simulink model "ACC_Project"  (R2020a)
settings: Solver=FixedStepDiscrete  StartTime=0.0  StopTime=10.0  FixedStep=0.01  RelTol=1e-3
settings Model: DataDictionary=ACC_Project_SLDD.sldd  EnableAccessToBaseWorkspace=off  Creator=todka  LastModifiedBy=todka
settings OptimizationCC: DefaultParameterBehavior=Inlined  EnhancedBackFolding=on  PassReuseOutputArgsAs=Individual arguments  ZeroExternalMemoryAtStartup=off  ZeroInternalMemoryAtStartup=off  OptimizeBlockOrder=speed  DifferentSizesBufferReuse=on  OptimizationCustomize=off  EfficientTunableParamExpr=on
settings DebuggingCC: SignalInfNanChecking=error  CheckMatrixSingularityMsg=error  IntegerOverflowMsg=error  ParameterTunabilityLossMsg=error  UniqueDataStoreMsg=error  StrictBusMsg=ErrorOnBusTreatedAsVector  IntegerSaturationMsg=error
settings SFSimCC: MATLABDynamicMemAlloc=off
settings RTWCC: SystemTargetFile=ert.tlc  TemplateMakefile=ert_default_tmf  GenerateReport=on
settings CodeAppCC: ForceParamTrailComments=on  IgnoreCustomStorageClasses=off  OperatorAnnotations=on  SimulinkDataObjDesc=on  SFDataObjDesc=on  InsertBlockDesc=on
settings ERTTargetCC: TargetLangStandard=C99 (ISO)  GenerateSampleERTMain=on  InlinedParameterPlacement=NonHierarchical  ERTCustomFileTemplate=example_file_process.tlc
settings ConfigComp: CovMetricSettings=dcmwe

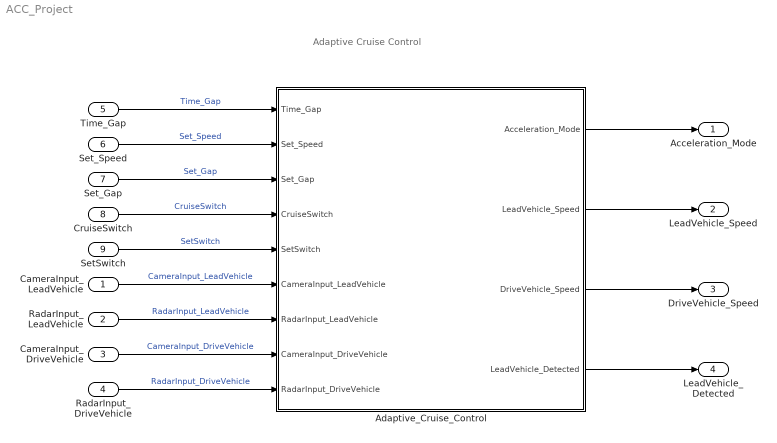
== system ACC_Project ==
  note: Adaptive Cruise Control
  CameraInput_LeadVehicle : Inport
  RadarInput_LeadVehicle : Inport  Port=2
  CameraInput_DriveVehicle : Inport  Port=3
  RadarInput_DriveVehicle : Inport  Port=4
  Time_Gap : Inport  Port=5
  Set_Speed : Inport  Port=6
  Set_Gap : Inport  Port=7
  CruiseSwitch : Inport  Port=8
  SetSwitch : Inport  Port=9
  Adaptive_Cruise_Control : Subsystem
  Acceleration_Mode : Outport
  LeadVehicle_Speed : Outport  Port=2
  DriveVehicle_Speed : Outport  Port=3
  LeadVehicle_Detected : Outport  Port=4
  wires:
  Time_Gap/1 -> Adaptive_Cruise_Control/1(Time_Gap)  "Time_Gap"
  Set_Speed/1 -> Adaptive_Cruise_Control/2(Set_Speed)  "Set_Speed"
  Set_Gap/1 -> Adaptive_Cruise_Control/3(Set_Gap)  "Set_Gap"
  CruiseSwitch/1 -> Adaptive_Cruise_Control/4(CruiseSwitch)  "CruiseSwitch"
  SetSwitch/1 -> Adaptive_Cruise_Control/5(SetSwitch)  "SetSwitch"
  CameraInput_LeadVehicle/1 -> Adaptive_Cruise_Control/6(CameraInput_LeadVehicle)  "CameraInput_LeadVehicle"
  RadarInput_LeadVehicle/1 -> Adaptive_Cruise_Control/7(RadarInput_LeadVehicle)  "RadarInput_LeadVehicle"
  CameraInput_DriveVehicle/1 -> Adaptive_Cruise_Control/8(CameraInput_DriveVehicle)  "CameraInput_DriveVehicle"
  RadarInput_DriveVehicle/1 -> Adaptive_Cruise_Control/9(RadarInput_DriveVehicle)  "RadarInput_DriveVehicle"
  Adaptive_Cruise_Control/1(Acceleration_Mode) -> Acceleration_Mode/1
  Adaptive_Cruise_Control/2(LeadVehicle_Speed) -> LeadVehicle_Speed/1
  Adaptive_Cruise_Control/3(DriveVehicle_Speed) -> DriveVehicle_Speed/1
  Adaptive_Cruise_Control/4(LeadVehicle_Detected) -> LeadVehicle_Detected/1

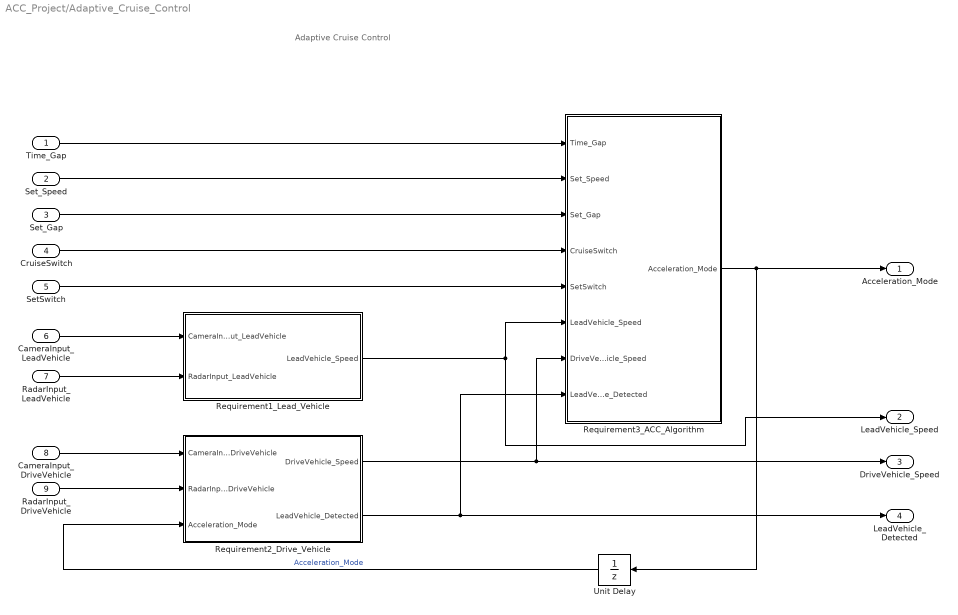
== system ACC_Project/Adaptive_Cruise_Control ==
  note: Adaptive Cruise Control
  Time_Gap : Inport
  Set_Speed : Inport  Port=2
  Set_Gap : Inport  Port=3
  CruiseSwitch : Inport  Port=4
  SetSwitch : Inport  Port=5
  CameraInput_LeadVehicle : Inport  Port=6
  RadarInput_LeadVehicle : Inport  Port=7
  CameraInput_DriveVehicle : Inport  Port=8
  RadarInput_DriveVehicle : Inport  Port=9
  Requirement1_Lead_Vehicle : Subsystem
  Requirement2_Drive_Vehicle : Subsystem
  Requirement3_ACC_Algorithm : Subsystem
  Unit Delay : UnitDelay  SampleTime=-1  HasFrameUpgradeWarning=on
  Acceleration_Mode : Outport
  LeadVehicle_Speed : Outport  Port=2
  DriveVehicle_Speed : Outport  Port=3
  LeadVehicle_Detected : Outport  Port=4
  wires:
  Requirement2_Drive_Vehicle/2(LeadVehicle_Detected) -> Requirement3_ACC_Algorithm/8(LeadVehicle_Detected), LeadVehicle_Detected/1
  CruiseSwitch/1 -> Requirement3_ACC_Algorithm/4(CruiseSwitch)
  Requirement1_Lead_Vehicle/1(LeadVehicle_Speed) -> LeadVehicle_Speed/1, Requirement3_ACC_Algorithm/6(LeadVehicle_Speed)
  SetSwitch/1 -> Requirement3_ACC_Algorithm/5(SetSwitch)
  Time_Gap/1 -> Requirement3_ACC_Algorithm/1(Time_Gap)
  Set_Gap/1 -> Requirement3_ACC_Algorithm/3(Set_Gap)
  RadarInput_LeadVehicle/1 -> Requirement1_Lead_Vehicle/2(RadarInput_LeadVehicle)
  Set_Speed/1 -> Requirement3_ACC_Algorithm/2(Set_Speed)
  Requirement2_Drive_Vehicle/1(DriveVehicle_Speed) -> DriveVehicle_Speed/1, Requirement3_ACC_Algorithm/7(DriveVehicle_Speed)
  CameraInput_DriveVehicle/1 -> Requirement2_Drive_Vehicle/1(CameraInput_DriveVehicle)
  CameraInput_LeadVehicle/1 -> Requirement1_Lead_Vehicle/1(CameraInput_LeadVehicle)
  RadarInput_DriveVehicle/1 -> Requirement2_Drive_Vehicle/2(RadarInput_DriveVehicle)
  Requirement3_ACC_Algorithm/1(Acceleration_Mode) -> Unit Delay/1, Acceleration_Mode/1
  Unit Delay/1 -> Requirement2_Drive_Vehicle/3(Acceleration_Mode)  "Acceleration_Mode"

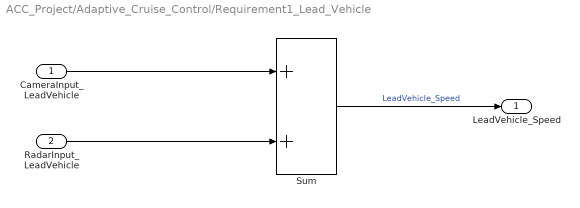
== system ACC_Project/Adaptive_Cruise_Control/Requirement1_Lead_Vehicle ==
  CameraInput_LeadVehicle : Inport
  RadarInput_LeadVehicle : Inport  Port=2
  Sum : Sum
  LeadVehicle_Speed : Outport
  wires:
  RadarInput_LeadVehicle/1 -> Sum/2
  CameraInput_LeadVehicle/1 -> Sum/1
  Sum/1 -> LeadVehicle_Speed/1  "LeadVehicle_Speed"

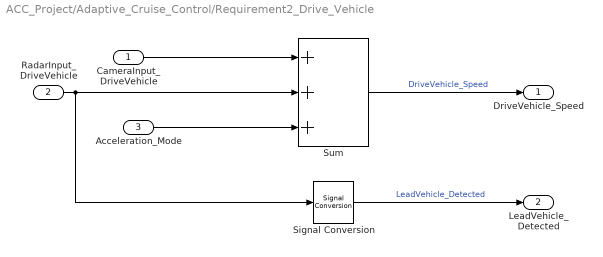
== system ACC_Project/Adaptive_Cruise_Control/Requirement2_Drive_Vehicle ==
  CameraInput_DriveVehicle : Inport
  RadarInput_DriveVehicle : Inport  Port=2
  Acceleration_Mode : Inport  Port=3
  Signal Conversion : SignalConversion  OverrideOpt=off
  Sum : Sum  Inputs=+++
  DriveVehicle_Speed : Outport
  LeadVehicle_Detected : Outport  Port=2
  wires:
  RadarInput_DriveVehicle/1 -> Signal Conversion/1, Sum/2
  CameraInput_DriveVehicle/1 -> Sum/1
  Sum/1 -> DriveVehicle_Speed/1  "DriveVehicle_Speed"
  Signal Conversion/1 -> LeadVehicle_Detected/1  "LeadVehicle_Detected"
  Acceleration_Mode/1 -> Sum/3

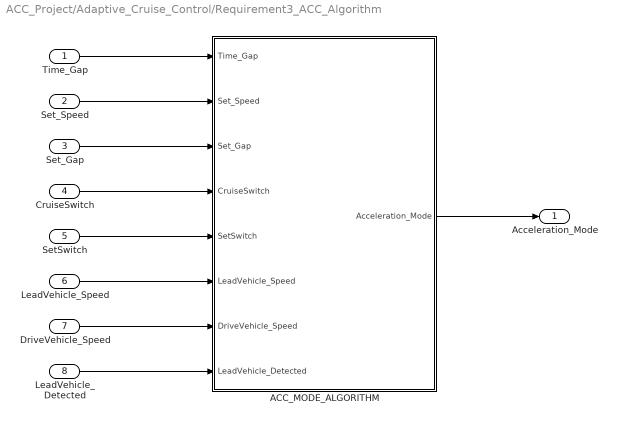
== system ACC_Project/Adaptive_Cruise_Control/Requirement3_ACC_Algorithm ==
  Time_Gap : Inport
  Set_Speed : Inport  Port=2
  Set_Gap : Inport  Port=3
  CruiseSwitch : Inport  Port=4
  SetSwitch : Inport  Port=5
  LeadVehicle_Speed : Inport  Port=6
  DriveVehicle_Speed : Inport  Port=7
  LeadVehicle_Detected : Inport  Port=8
  ACC_MODE_ALGORITHM : Stateflow chart  TreatAsAtomicUnit=on
  Acceleration_Mode : Outport
  wires:
  Time_Gap/1 -> ACC_MODE_ALGORITHM/1(Time_Gap)
  Set_Speed/1 -> ACC_MODE_ALGORITHM/2(Set_Speed)
  Set_Gap/1 -> ACC_MODE_ALGORITHM/3(Set_Gap)
  CruiseSwitch/1 -> ACC_MODE_ALGORITHM/4(CruiseSwitch)
  SetSwitch/1 -> ACC_MODE_ALGORITHM/5(SetSwitch)
  LeadVehicle_Speed/1 -> ACC_MODE_ALGORITHM/6(LeadVehicle_Speed)
  DriveVehicle_Speed/1 -> ACC_MODE_ALGORITHM/7(DriveVehicle_Speed)
  LeadVehicle_Detected/1 -> ACC_MODE_ALGORITHM/8(LeadVehicle_Detected)
  ACC_MODE_ALGORITHM/1(Acceleration_Mode) -> Acceleration_Mode/1

== stateflow chart ACC_Project/Adaptive_Cruise_Control/Requirement3_ACC_Algorithm/ACC_MODE_ALGORITHM ==
  state ACC_OFF_MODE
    entry:
    Acceleration_Mode=0;
  state ACC_STANDBY_MODE
    entry:
    Acceleration_Mode=1;
  state ACC_ON_MODE
    state LeadVehicle_Detected_Follow
      Acceleration_Mode=2;
    state LeadVehicle_Detected_Resume
      Acceleration_Mode=3;
    state LeadVehicle_Not_Detected_Resume
      Acceleration_Mode=1;
    state LeadVehicle_Not_Detected
      Acceleration_Mode=1;
    state LeadVehicle_Speed_equal_Set_Speed
      Acceleration_Mode=5;
    state LeadVehicle_Speed_lessthan_Set_Speed
      Acceleration_Mode=4;
    (default) -> LeadVehicle_Detected_Follow
    LeadVehicle_Detected_Resume -> LeadVehicle_Detected_Follow [order 1] : [(DriveVehicle_Speed == Set_Speed) && ...
        | (LeadVehicle_Speed >= Set_Speed) && ...
        | (Time_Gap >= Set_Gap)]
    LeadVehicle_Detected_Resume -> LeadVehicle_Not_Detected_Resume [order 3] : [LeadVehicle_Detected==0]
    LeadVehicle_Detected_Follow -> LeadVehicle_Not_Detected [order 1] : [LeadVehicle_Detected == 0]
    LeadVehicle_Speed_equal_Set_Speed -> LeadVehicle_Detected_Resume [order 1] : [(DriveVehicle_Speed < Set_Speed) && ...
        | (LeadVehicle_Speed > DriveVehicle_Speed) || ...
        | (Time_Gap >= Set_Gap)]
    LeadVehicle_Detected_Resume -> LeadVehicle_Speed_equal_Set_Speed [order 2] : [(DriveVehicle_Speed < Set_Speed) && ...
        | (LeadVehicle_Speed > DriveVehicle_Speed) && ...
        | (Time_Gap >= Set_Gap)]
    LeadVehicle_Speed_equal_Set_Speed -> LeadVehicle_Not_Detected_Resume [order 3] : [(LeadVehicle_Detected == 0) || ...
        | (DriveVehicle_Speed <= Set_Speed)]
    LeadVehicle_Not_Detected -> LeadVehicle_Detected_Follow [order 2] : [(LeadVehicle_Detected==1) && ...
        | (DriveVehicle_Speed == Set_Speed) && ...
        | (LeadVehicle_Speed >= Set_Speed) && ...
        | (Time_Gap >= Set_Gap)]
    LeadVehicle_Detected_Follow -> LeadVehicle_Speed_lessthan_Set_Speed [order 2] : [(LeadVehicle_Detected == 1) && ...
        | (LeadVehicle_Speed < Set_Speed) ||...
        |  (Time_Gap < Set_Gap)]
    LeadVehicle_Speed_lessthan_Set_Speed -> LeadVehicle_Not_Detected [order 1] : [(LeadVehicle_Detected == 0) &&...
        |  (DriveVehicle_Speed == Set_Speed)]
    LeadVehicle_Not_Detected -> LeadVehicle_Speed_lessthan_Set_Speed [order 1] : [(LeadVehicle_Detected == 1) && ...
        | (LeadVehicle_Speed < Set_Speed) || ...
        | (Time_Gap < Set_Gap)]
    LeadVehicle_Speed_equal_Set_Speed -> LeadVehicle_Speed_lessthan_Set_Speed [order 2] : [(LeadVehicle_Speed<Set_Speed) && ...
        | (LeadVehicle_Speed<DriveVehicle_Speed) || ...
        | (Time_Gap == 0.75*Set_Gap)]
    LeadVehicle_Speed_lessthan_Set_Speed -> LeadVehicle_Speed_equal_Set_Speed [order 2] : [((LeadVehicle_Speed*1.25>=DriveVehicle_Speed) && ...
        | (LeadVehicle_Speed * 0.75<=DriveVehicle_Speed)) && ...
        | (DriveVehicle_Speed < Set_Speed) && ...
        | ((Time_Gap<=1.25*Set_Gap) && (Time_Gap >=0.75*Set_Gap))]
  (default) -> ACC_OFF_MODE
  ACC_OFF_MODE -> ACC_STANDBY_MODE : [CruiseSwitch==1]
  ACC_STANDBY_MODE -> ACC_OFF_MODE [order 1] : [CruiseSwitch==0]
  ACC_ON_MODE -> ACC_OFF_MODE [order 1] : [CruiseSwitch==0]
  ACC_ON_MODE -> ACC_STANDBY_MODE [order 2] : [SetSwitch==0]
  ACC_STANDBY_MODE -> ACC_ON_MODE [order 2] : [SetSwitch==1]
  data: Acceleration_Mode output; Time_Gap input; Set_Speed input; Set_Gap input; CruiseSwitch input; SetSwitch input; LeadVehicle_Speed input; DriveVehicle_Speed input; LeadVehicle_Detected input
